simulink model "Sliding_Window_Second_Order"  (R2021a)
settings: Solver=FixedStepAuto  StartTime=0.0  StopTime=10.0  FixedStep=0.005  RelTol=1e-3
model workspace (MAT data in the model file):
  Kp = 1500
  N = 45
  Nd = 40
  Td = 0.0065
  Ts = 0.005
  alpha = 1.3
settings Model: Creator=Henrique Mesquita  LastModifiedBy=Henrique Mesquita
settings DataIOCC: SaveOutput=off  SaveTime=off

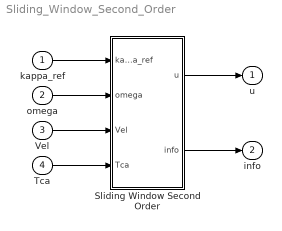
== system Sliding_Window_Second_Order ==
  kappa_ref : Inport  OutDataTypeStr=double  PortDimensions=1  SampleTime=[0.0050000000000000001,0]
  omega : Inport  Port=2  OutDataTypeStr=double  PortDimensions=1  SampleTime=[0.0050000000000000001,0]
  Vel : Inport  Port=3  OutDataTypeStr=double  PortDimensions=1  SampleTime=[0.0050000000000000001,0]
  Tca : Inport  Port=4  OutDataTypeStr=double  PortDimensions=1  SampleTime=[0.0050000000000000001,0]
  Sliding Window Second Order : MATLAB Function  TreatAsAtomicUnit=on  VariantControl=Choice
  u : Outport  OutDataTypeStr=double  PortDimensions=1  SampleTime=[0.0050000000000000001,0]
  info : Outport  Port=2  OutDataTypeStr=Bus: control_info_bus  PortDimensions=1  SampleTime=[0.0050000000000000001,0]  BusOutputAsStruct=on
  wires:
  kappa_ref/1 -> Sliding Window Second Order/1(kappa_ref)
  omega/1 -> Sliding Window Second Order/2(omega)
  Vel/1 -> Sliding Window Second Order/3(Vel)
  Tca/1 -> Sliding Window Second Order/4(Tca)
  Sliding Window Second Order/1(u) -> u/1
  Sliding Window Second Order/2(info) -> info/1

== matlab function Sliding_Window_Second_Order/Sliding Window Second Order ==
  data: kappa_ref input; u output; omega input; Vel input; Tca input; info output Bus: control_info_bus; Kp parameter; Td parameter; Ts parameter; alpha parameter; N parameter; Nd parameter
function [u,info] = fcn(kappa_ref, omega, Vel, Tca, Kp, Td, Ts, alpha, N, Nd)

%%% Definition of persistent variables
persistent u_mem;
persistent kappa_mem;
persistent e_ant;
persistent ud_ant;
persistent k_ref_ant;
persistent phi;
persistent alpha_chap;
persistent s_y;
persistent s_u;

%%% Initialization of the persistent values
if (isempty(u_mem)||isempty(kappa_mem)||isempty(k_ref_ant)||isempty(phi)||isempty(alpha_chap)||isempty(s_y)||isempty(s_u))
    
    %%% Initial allocation of the persistent variables
    phi = 0;
    alpha_chap = alpha;
    u_mem = zeros(1,N+1);
    kappa_mem = zeros(1,N+1);
    k_ref_ant = kappa_ref;
    e_ant = 0;
    ud_ant = 0;
    
    %%% Early calculation and saving of the algebraic estimator coefficients
    T = N*Ts;
    i = N-1:-1:1;
    s_y = 60/T^5*[Ts/2*(T^2-6*T*N*Ts+6*(N*Ts)^2), Ts*(T^2-6*T*i*Ts+6*(i*Ts).^2), Ts/2*(T^2-6*0*N*Ts+6*(0*Ts)^2)];
    s_u = -30/T^5*[Ts/2*(T-N*Ts)^2*(N*Ts)^2, Ts*(T-i*Ts).^2.*(i*Ts).^2, Ts/2*(T-0*Ts)^2*(0*Ts)^2];
end

%%% Parameter transformations and definitions
omega = omega*2*pi/60;
Vel = Vel/3.6;
re = 0.284;
Iw = 0.8;

%%% Slip and error estimation
dot_yd = (kappa_ref - k_ref_ant) / Ts;
kappa = (omega*re-Vel)/(max([Vel 3/3.6]));
e = kappa-kappa_ref;

%%% Control signal calculation
% ud = Kp*Td/Ts*(kappa-kappa_mem(1));
% ud = Td/(Td+Nd*Ts)*ud_ant + Kp*Nd*Td/(Td+Nd*Ts)*(e - e_ant);
ud = Td/(Td+Nd*Ts)*ud_ant + Kp*Nd*Td/(Td+Nd*Ts)*(kappa-kappa_mem(1));
du = (-phi+dot_yd-Kp*e-ud)/alpha_chap;
% ud = 0;
% du = (-phi+dot_yd-Kp*e)/alpha_chap;

%%% Saturation of the control signal
if(du>0)
    du = 0;
elseif (du<-Tca)
    du = -Tca;
end

%%% Block outputs
% u = du+Tca;
u = du;
info = struct('Phi',phi,'kappa',kappa,'u',u,'du',du,'e',e,'a',alpha_chap,'ui',0,'ud',ud,'state',0);

%%% Memory actualization
for i = 0:N-1
    u_mem(N+1-i) = u_mem(N-i);
    kappa_mem(N+1-i) = kappa_mem(N-i);
end
u_mem(1) = du;
kappa_mem(1) = kappa;
e_ant = e;
ud_ant = ud;
k_ref_ant = kappa_ref;
alpha_chap = max([0.01,min([alpha,re/(Iw*max([Vel 0.001]))])]);
% alpha_chap = alpha;

%%% Algebraic Estimation
phi=0;
for i=1:N+1
    phi = phi + s_y(i)*kappa_mem(i) + alpha_chap*s_u(i)*u_mem(i);
end
